simulink model "Banco_Capacitores_Automatico"  (R2022a)
settings: Solver=ode14x  StartTime=0.0  StopTime=1  FixedStep=5e-5  RelTol=1e-3
undefined symbols (not defined in the file): D11, Delta
libraries: spsSeriesRLCBranchLib x24, spsParallelRLCLoadLib x21, spsGroundLib x11, spsThreePhaseBreakerLib x7, spsLinearTransformerLib x6, spsCurrentMeasurementLib x4, spsVoltageMeasurementLib x3, eeRmsMeasurement x2, spsPower3phInstantaneousLib x2, spsThreePhaseVIMeasurementLib x2, spsThreePhaseSourceLib x1, spsRMSLib x1
settings Model: Creator=Luiz  LastModifiedBy=Luiz

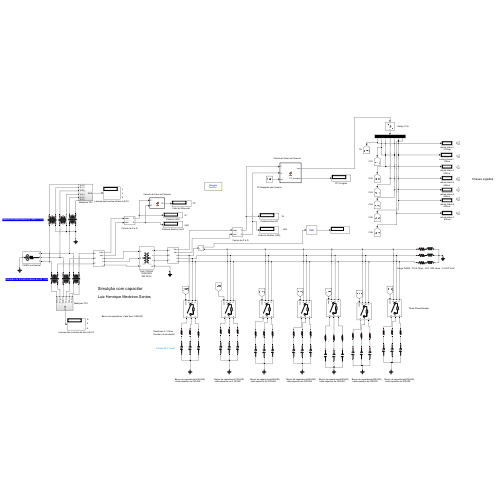
[thumbnail: Simulink's stored preview of the top-level diagram]
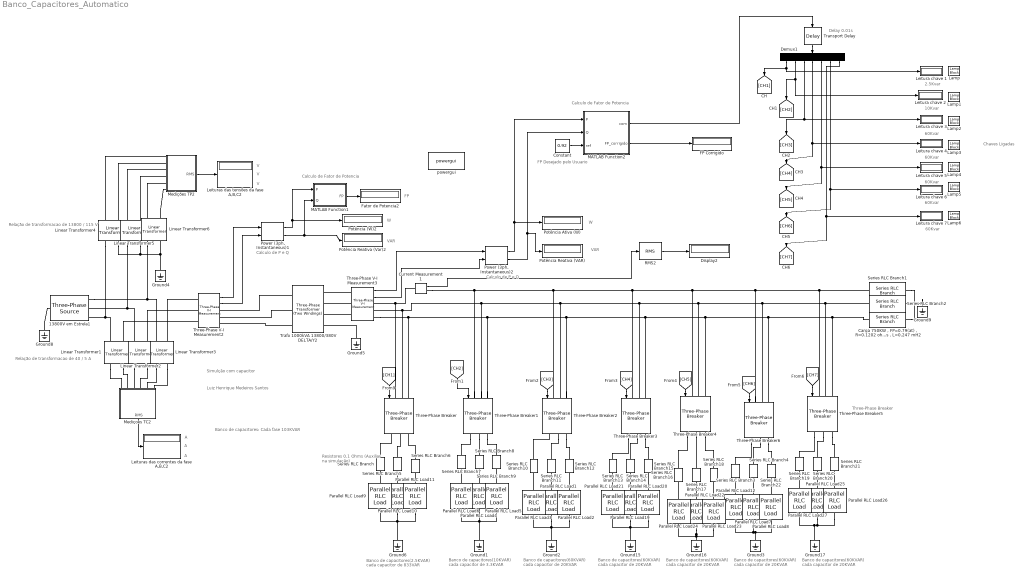
== system Banco_Capacitores_Automatico ==
  note: Three-Phase Breaker
  note: Banco de capacitores(2.5KVAR)
      |  cada capacitor de 833VAR
  note: Chaves Ligadas
  note: FP Desejado pelo Usuario
  note: 2.5Kvar
  note: Delay 0.01s
  note: Resistores 0.1 Ohms
      | (Auxiliar na simulação)
  note: A
  note: Simulção com capacitor
  note: Calculo de P e Q
  note: A
  note: V
  note: Luiz Henrique Medeiros Santos
  note: Relação de transformacao de 40 / 5 A
  note: V
  note: VAR
  note: FP
  note: Calculo de Fator de Potencia
  note: A
  note: V
  note: Calculo de P e Q
  note: Banco de capacitores: Cada fase 103KVAR
  note: VAR
  note: Relação de transformacao de 13800 / 115 V
  note: W
  note: Calculo de Fator de Potencia
  note: W
  note: 10Kvar
  note: 60Kvar
  note: 60Kvar
  note: 60Kvar
  note: 60Kvar
  note: 60Kvar
  note: Banco de capacitores(10KVAR)
      |  cada capacitor de 3.3KVAR
  note: Banco de capacitores(60KVAR)
      |  cada capacitor de 20KVAR
  note: Banco de capacitores(60KVAR)
      |  cada capacitor de 20KVAR
  note: Banco de capacitores(60KVAR)
      |  cada capacitor de 20KVAR
  note: Banco de capacitores(60KVAR)
      |  cada capacitor de 20KVAR
  note: Banco de capacitores(60KVAR)
      |  cada capacitor de 20KVAR
  13800V em Estrela1 : spsThreePhaseSourceLib/Three-Phase Source  InternalConnection=Yn  VoltagePhases=off  Voltage=13800  PhaseAngle=0  Voltage_phases=[25e3 25e3 25e3]/sqrt(3)  PhaseAngles_phases=[0 -120 +120]  Frequency=60  NonIdealSource=on  SpecifyImpedance=off  Resistance=0.0001  Inductance=0  ShortCircuitLevel=100e6  BaseVoltage=0  XRratio=7  BusType=swing  Pref=10e3  Qref=0  Prefabc=[10e3, 10e3, 10e3]  Qrefabc=[0, 0, 0]  Qmin=-inf  Qmax=inf
  "Carga 750KW , FP=0.79(at) , R=0.1202 ohms , L=0,247 mH2" : spsSeriesRLCBranchLib/Series RLC Branch  LConnTagsString=__new0  RConnTagsString=__new0  BranchType=RL  Resistance=0.1202  Inductance=0.247e-3  SetiL0=off  InitialCurrent=0  Capacitance=0  Setx0=off  InitialVoltage=0  Measurements=None
  Constant : Constant  Value=0.92
  Current Measurement1 : spsCurrentMeasurementLib/Current Measurement  PhasorSimulation=off  OutputType=Complex  PSBequivalent=0
  Demux1 : Demux  Outputs=7
  Display2 : Display
  FP Corrigido : Display
      settings: Format=bank
  Fator de Potencia2 : Display
      settings: Format=bank
  Ground{1..6,8..9,15..17} (11 alike) : spsGroundLib/Ground  LConnTagsString=a
  Lamp{,1..6} (7 alike) : LampBlock  LabelPosition=Hide
  Leitura chave {1..7} (7 alike) : Display
  Leituras das correntes da fase A,B,C2 : Display
      settings: Format=bank
  Leituras das tensões da fase A,B,C2 : Display
      settings: Format=bank
  Linear Transformer1 : spsLinearTransformerLib/Linear Transformer  UNITS=pu  NominalPower=[ 500 60 ]  winding1="[ 1 0.002  0.08 ]"  winding2="[ 8  0.002  0.08 ]"  ThreeWindings=off  winding3=[ 315e3 0.002 0.08 ]  RmLm=[ 500 500 ]  Measurements=None  DataType=off
  Linear Transformer2 : spsLinearTransformerLib/Linear Transformer  UNITS=pu  NominalPower=[ 500 60 ]  winding1="[ 1 0.002  0.08 ]"  winding2="[ 8  0.002  0.08 ]"  ThreeWindings=off  winding3=[ 315e3 0.002 0.08 ]  RmLm=[ 500 500 ]  Measurements=None  DataType=off
  Linear Transformer3 : spsLinearTransformerLib/Linear Transformer  UNITS=pu  NominalPower=[ 500 60 ]  winding1="[ 1 0.002  0.08 ]"  winding2="[ 8  0.002  0.08 ]"  ThreeWindings=off  winding3=[ 315e3 0.002 0.08 ]  RmLm=[ 500 500 ]  Measurements=None  DataType=off
  Linear Transformer4 : spsLinearTransformerLib/Linear Transformer  UNITS=pu  NominalPower=[ 500 60 ]  winding1="[ 7970 0.002  0.08 ]"  winding2="[ 115  0.002  0.08 ]"  ThreeWindings=off  winding3=[ 315e3 0.002 0.08 ]  RmLm=[ 500 500 ]  Measurements=None  DataType=off
  Linear Transformer5 : spsLinearTransformerLib/Linear Transformer  UNITS=pu  NominalPower=[ 500 60 ]  winding1="[ 7970 0.002  0.08 ]"  winding2="[ 115  0.002  0.08 ]"  ThreeWindings=off  winding3=[ 315e3 0.002 0.08 ]  RmLm=[ 500 500 ]  Measurements=None  DataType=off
  Linear Transformer6 : spsLinearTransformerLib/Linear Transformer  UNITS=pu  NominalPower=[ 500 60 ]  winding1="[ 7970 0.002  0.08 ]"  winding2="[ 115  0.002  0.08 ]"  ThreeWindings=off  winding3=[ 315e3 0.002 0.08 ]  RmLm=[ 500 500 ]  Measurements=None  DataType=off
  MATLAB Function1 : MATLAB Function  TreatAsAtomicUnit=on
  MATLAB Function2 : MATLAB Function  TreatAsAtomicUnit=on  SystemSampleTime=1
  Mediçoes TC2 : Subsystem
  Medições TP2 : Subsystem
  Parallel RLC Load{1,3,7..8,12,19..27} (14 alike) : spsParallelRLCLoadLib/Parallel RLC Load  LConnTagsString=a  RConnTagsString=__new0  NominalVoltage=217.78  NominalFrequency=60  ActivePower=0  InductivePower=0  CapacitivePower=20e3  Setx0=off  InitialVoltage=0  SetiL0=off  InitialCurrent=0  Measurements=None  LoadType=constant Z
      settings: AttributesFormatString=\n  SourceProductBaseCode=PS
  Parallel RLC Load10 : spsParallelRLCLoadLib/Parallel RLC Load  LConnTagsString=a  RConnTagsString=__new0  NominalVoltage=217.78  NominalFrequency=60  ActivePower=0  InductivePower=0  CapacitivePower=0.833e3  Setx0=off  InitialVoltage=0  SetiL0=off  InitialCurrent=0  Measurements=None  LoadType=constant Z
      settings: AttributesFormatString=\n  SourceProductBaseCode=PS
  Parallel RLC Load11 : spsParallelRLCLoadLib/Parallel RLC Load  LConnTagsString=a  RConnTagsString=__new0  NominalVoltage=217.78  NominalFrequency=60  ActivePower=0  InductivePower=0  CapacitivePower=0.833e3  Setx0=off  InitialVoltage=0  SetiL0=off  InitialCurrent=0  Measurements=None  LoadType=constant Z
      settings: AttributesFormatString=\n  SourceProductBaseCode=PS
  Parallel RLC Load2 : spsParallelRLCLoadLib/Parallel RLC Load  LConnTagsString=a  RConnTagsString=__new0  NominalVoltage=217.78  NominalFrequency=60  ActivePower=0  InductivePower=0  CapacitivePower=20e3  Setx0=off  InitialVoltage=0  SetiL0=on  InitialCurrent=0  Measurements=None  LoadType=constant Z
      settings: AttributesFormatString=\n  SourceProductBaseCode=PS
  Parallel RLC Load4 : spsParallelRLCLoadLib/Parallel RLC Load  LConnTagsString=a  RConnTagsString=__new0  NominalVoltage=217.78  NominalFrequency=60  ActivePower=0  InductivePower=0  CapacitivePower=3.33e3  Setx0=off  InitialVoltage=0  SetiL0=off  InitialCurrent=0  Measurements=None  LoadType=constant Z
      settings: AttributesFormatString=\n  SourceProductBaseCode=PS
  Parallel RLC Load5 : spsParallelRLCLoadLib/Parallel RLC Load  LConnTagsString=a  RConnTagsString=__new0  NominalVoltage=217.78  NominalFrequency=60  ActivePower=0  InductivePower=0  CapacitivePower=3.33e3  Setx0=off  InitialVoltage=0  SetiL0=off  InitialCurrent=0  Measurements=None  LoadType=constant Z
      settings: AttributesFormatString=\n  SourceProductBaseCode=PS
  Parallel RLC Load6 : spsParallelRLCLoadLib/Parallel RLC Load  LConnTagsString=a  RConnTagsString=__new0  NominalVoltage=217.78  NominalFrequency=60  ActivePower=0  InductivePower=0  CapacitivePower=3.33e3  Setx0=off  InitialVoltage=0  SetiL0=off  InitialCurrent=0  Measurements=None  LoadType=constant Z
      settings: AttributesFormatString=\n  SourceProductBaseCode=PS
  Parallel RLC Load9 : spsParallelRLCLoadLib/Parallel RLC Load  LConnTagsString=a  RConnTagsString=__new0  NominalVoltage=217.78  NominalFrequency=60  ActivePower=0  InductivePower=0  CapacitivePower=0.833e3  Setx0=off  InitialVoltage=0  SetiL0=off  InitialCurrent=0  Measurements=None  LoadType=constant Z
      settings: AttributesFormatString=\n  SourceProductBaseCode=PS
  Potência (W)2 : Display
      settings: Format=bank
  Potência Ativa (W) : Display
      settings: Format=bank
  Potência Reativa (VAR) : Display
      settings: Format=bank
  Potência Reativa (Var)2 : Display
      settings: Format=bank
  "Power (3ph, Instantaneous)1" : spsPower3phInstantaneousLib/Power (3ph, Instantaneous)
  "Power (3ph, Instantaneous)2" : spsPower3phInstantaneousLib/Power (3ph, Instantaneous)
  RMS2 : spsRMSLib/RMS  TrueRMS=on  Freq=60  RMSInit=120  Ts=0
  Series RLC Branch{,3..22} (21 alike) : spsSeriesRLCBranchLib/Series RLC Branch  LConnTagsString=__new0  RConnTagsString=__new0  BranchType=R  Resistance=0.05  Inductance=0  SetiL0=off  InitialCurrent=0  Capacitance=0  Setx0=off  InitialVoltage=0  Measurements=None
  Series RLC Branch1 : spsSeriesRLCBranchLib/Series RLC Branch  LConnTagsString=__new0  RConnTagsString=__new0  BranchType=RL  Resistance=0.1202  Inductance=0.247e-3  SetiL0=off  InitialCurrent=0  Capacitance=0  Setx0=off  InitialVoltage=0  Measurements=None
  Series RLC Branch2 : spsSeriesRLCBranchLib/Series RLC Branch  LConnTagsString=__new0  RConnTagsString=__new0  BranchType=RL  Resistance=0.1202  Inductance=0.247e-3  SetiL0=off  InitialCurrent=0  Capacitance=0  Setx0=off  InitialVoltage=0  Measurements=None
  Three-Phase V-I Measurement2 : spsThreePhaseVIMeasurementLib/Three-Phase V-I Measurement  VoltageMeasurement=phase-to-ground  SetLabelV=off  LabelV=Vabc  Vpu=off  VpuLL=off  CurrentMeasurement=yes  SetLabelI=off  LabelI=Iabc  Ipu=off  Pbase=100e6  Vbase=500e3  OutputType=Complex  PhasorSimulation=off  PSBequivalent=0
  Three-Phase V-I Measurement3 : spsThreePhaseVIMeasurementLib/Three-Phase V-I Measurement  VoltageMeasurement=phase-to-ground  SetLabelV=off  LabelV=Vabc  Vpu=off  VpuLL=off  CurrentMeasurement=yes  SetLabelI=off  LabelI=Iabc  Ipu=off  Pbase=100e6  Vbase=500e3  OutputType=Complex  PhasorSimulation=off  PSBequivalent=0
  Three-Phase Breaker{,1..6} (7 alike) : spsThreePhaseBreakerLib/Three-Phase Breaker  InitialState=open  SwitchA=on  SwitchB=on  SwitchC=on  SwitchTimes="[1/60  5/60]"  External=on  BreakerResistance=0.01  SnubberResistance=1e6  SnubberCapacitance=inf  Measurements=None
  Trafo 1000kVA 13800/380V DELTA/Y2 : spsThreePhaseTransformerTwoWindingsLib/Three-Phase Transformer (Two Windings)  Winding1Connection=Delta (D11)  Winding2Connection=Yn  CoreType=Three single-phase transformers  SetSaturation=off  Hysteresis=off  DataFile='hysteresis'  SetInitialFlux=off  Measurements=None  UNITS=SI  NominalPower=[ 1e6 , 60 ]  Winding1=[13800 0.0001 0.0001]  Winding2=[380 0.00001 1e-05]  Rm=2.8566e+06  Lm=757.74  L0=0.5  Saturation=[0 0;0.081983 62.122;34.16 78.688]  InitialFluxes=[ 0.8 , -0.8 , 0.7 ]  BreakLoop=off  DiscreteSolver=Trapezoidal iterative  DataType=on  TransfoNumber=1
  Transport Delay : TransportDelay  DelayTime=0.1  BufferSize=10240
  powergui : spspowerguiLib/powergui  Priority=1  SimulationMode=Discrete  SampleTime=50e-6  frequency=60  Iterations=50  frequencyindice=60  Pbase=100e6  ErrMax=1e-4  UnitsV=kV  UnitsW=MW  buscounter=0  FunctionMessages=off  echomessages=off  EnableUseOfTLC=off  CurrentSourceSwitches=off  DisableSnubberDevices=off  DisableRonSwitches=off  DisableVfSwitches=off  DisplayEquations=off  AutomaticDiscreteSolvers=off  SolverType=Tustin/Backward Euler (TBE)  Interpol=off  ExternalGateDelay=off  methode=off  Ts=100  x0status=blocks  SPID=on  SwTol=0  HookPort=off  NonlinearTolerance=1e-4  nMaxIteration=100  ContinueOnMaxIteration=off  RestoreLinks=warning  ResistiveCurrentMeasurement=off  Frange=[0:2:500]  Ylog=off  Xlog=on  ShowGrid=off  save=off  variable=ZData  structure=0  ZoomFFT=off  StartTime=0.0  cycles=1  DisplayStyle=1  fundamental=60  FreqAxis=off  MaxFrequency=1000  frequencyindicesteady=1  RmsSteady=1  display=off
  wires:
  "Power (3ph, Instantaneous)1"/1 -> MATLAB Function1/1(P), Potência (W)2/1
  Three-Phase V-I Measurement2/1 -> "Power (3ph, Instantaneous)1"/1
  Mediçoes TC2/1(RMS) -> Leituras das correntes da fase A,B,C2/1
  "Power (3ph, Instantaneous)1"/2 -> MATLAB Function1/2(Q), Potência Reativa (Var)2/1
  Three-Phase V-I Measurement3/2 -> "Power (3ph, Instantaneous)2"/2
  Current Measurement1/1 -> RMS2/1
  "Power (3ph, Instantaneous)2"/2 -> MATLAB Function2/2(Q), Potência Reativa (VAR)/1
  RMS2/1 -> Display2/1
  MATLAB Function2/2(FP_corrigido) -> FP Corrigido/1
  MATLAB Function1/1(FP) -> Fator de Potencia2/1
  Three-Phase V-I Measurement3/1 -> "Power (3ph, Instantaneous)2"/1
  Medições TP2/1(RMS) -> Leituras das tensões da fase A,B,C2/1
  "Power (3ph, Instantaneous)2"/1 -> MATLAB Function2/1(P), Potência Ativa (W)/1
  MATLAB Function2/1(com) -> Transport Delay/1
  Three-Phase V-I Measurement2/2 -> "Power (3ph, Instantaneous)1"/2
  Demux1/1 -> Leitura chave 1/1, [CH1]
  Demux1/2 -> Leitura chave 2/1, [CH2]
  Demux1/3 -> Leitura chave 3/1, [CH3]
  Demux1/4 -> [CH4], Leitura chave 4/1
  Demux1/5 -> [CH5], Leitura chave 5/1
  Demux1/6 -> [CH6], Leitura chave 6/1
  Demux1/7 -> [CH7], Leitura chave 7/1
  Constant/1 -> MATLAB Function2/3(ref)
  Transport Delay/1 -> Demux1/1
  [CH2] -> Three-Phase Breaker1/1
  [CH3] -> Three-Phase Breaker2/1
  [CH4] -> Three-Phase Breaker3/1
  [CH5] -> Three-Phase Breaker4/1
  [CH6] -> Three-Phase Breaker6/1
  [CH7] -> Three-Phase Breaker5/1
  [CH1] -> Three-Phase Breaker/1
  connections:
  Linear Transformer6/LConn1 -- Linear Transformer3/LConn1 -- 13800V em Estrela1/RConn1
  Linear Transformer2/LConn1 -- 13800V em Estrela1/RConn2 -- Linear Transformer5/LConn1
  Current Measurement1/LConn1 -- Three-Phase V-I Measurement3/RConn1 -- Three-Phase Breaker/LConn1
  Ground4/LConn1 -- Linear Transformer6/LConn2 -- Linear Transformer4/LConn2 -- Linear Transformer5/LConn2
  Series RLC Branch2/LConn1 -- Three-Phase Breaker6/LConn2 -- Three-Phase Breaker4/LConn2 -- Three-Phase Breaker3/LConn2 -- Three-Phase Breaker1/LConn2 -- Three-Phase V-I Measurement3/RConn2 -- Three-Phase Breaker/LConn2 -- Three-Phase Breaker2/LConn2 -- Three-Phase Breaker5/LConn2
  Parallel RLC Load9/RConn1 -- Parallel RLC Load11/RConn1 -- Ground6/LConn1 -- Parallel RLC Load10/RConn1
  Three-Phase V-I Measurement3/RConn3 -- Three-Phase Breaker1/LConn3 -- Three-Phase Breaker2/LConn3 -- Three-Phase Breaker3/LConn3 -- Three-Phase Breaker4/LConn3 -- Three-Phase Breaker6/LConn3 -- Three-Phase Breaker5/LConn3 -- "Carga 750KW , FP=0.79(at) , R=0.1202 ohms , L=0,247 mH2"/LConn1 -- Three-Phase Breaker/LConn3
  Linear Transformer4/LConn1 -- 13800V em Estrela1/RConn3 -- Linear Transformer1/LConn1
  Current Measurement1/RConn1 -- Three-Phase Breaker1/LConn1 -- Three-Phase Breaker3/LConn1 -- Three-Phase Breaker4/LConn1 -- Three-Phase Breaker6/LConn1 -- Three-Phase Breaker5/LConn1 -- Series RLC Branch1/LConn1 -- Three-Phase Breaker2/LConn1
  Three-Phase V-I Measurement3/LConn2 -- Trafo 1000kVA 13800/380V DELTA/Y2/RConn2
  Linear Transformer3/LConn2 -- Three-Phase V-I Measurement2/LConn1
  Three-Phase V-I Measurement3/LConn3 -- Trafo 1000kVA 13800/380V DELTA/Y2/RConn3
  Linear Transformer6/RConn2 -- Medições TP2/LConn6
  Ground8/LConn1 -- 13800V em Estrela1/LConn1
  Parallel RLC Load9/LConn1 -- Series RLC Branch/RConn1
  Trafo 1000kVA 13800/380V DELTA/Y2/LConn3 -- Three-Phase V-I Measurement2/RConn3
  Linear Transformer5/RConn2 -- Medições TP2/LConn4
  Linear Transformer2/RConn1 -- Mediçoes TC2/LConn3
  Linear Transformer6/RConn1 -- Medições TP2/LConn5
  Linear Transformer1/RConn1 -- Mediçoes TC2/LConn1
  Linear Transformer3/RConn2 -- Mediçoes TC2/LConn6
  Linear Transformer4/RConn2 -- Medições TP2/LConn2
  Trafo 1000kVA 13800/380V DELTA/Y2/LConn2 -- Three-Phase V-I Measurement2/RConn2
  Three-Phase V-I Measurement3/LConn1 -- Trafo 1000kVA 13800/380V DELTA/Y2/RConn1
  Trafo 1000kVA 13800/380V DELTA/Y2/LConn1 -- Three-Phase V-I Measurement2/RConn1
  Linear Transformer2/LConn2 -- Three-Phase V-I Measurement2/LConn2
  Parallel RLC Load10/LConn1 -- Series RLC Branch5/RConn1
  Linear Transformer1/RConn2 -- Mediçoes TC2/LConn2
  Linear Transformer3/RConn1 -- Mediçoes TC2/LConn5
  Linear Transformer5/RConn1 -- Medições TP2/LConn3
  Linear Transformer2/RConn2 -- Mediçoes TC2/LConn4
  Linear Transformer4/RConn1 -- Medições TP2/LConn1
  Linear Transformer1/LConn2 -- Three-Phase V-I Measurement2/LConn3
  Ground5/LConn1 -- Trafo 1000kVA 13800/380V DELTA/Y2/RConn4
  Series RLC Branch6/LConn1 -- Three-Phase Breaker/RConn3
  Ground9/LConn1 -- "Carga 750KW , FP=0.79(at) , R=0.1202 ohms , L=0,247 mH2"/RConn1 -- Series RLC Branch1/RConn1 -- Series RLC Branch2/RConn1
  Parallel RLC Load4/RConn1 -- Parallel RLC Load5/RConn1 -- Ground1/LConn1 -- Parallel RLC Load6/RConn1
  Parallel RLC Load4/LConn1 -- Series RLC Branch8/RConn1
  Parallel RLC Load6/LConn1 -- Series RLC Branch7/RConn1
  Parallel RLC Load5/LConn1 -- Series RLC Branch9/RConn1
  Parallel RLC Load1/RConn1 -- Parallel RLC Load2/RConn1 -- Ground2/LConn1 -- Parallel RLC Load3/RConn1
  Parallel RLC Load2/LConn1 -- Series RLC Branch12/RConn1
  Parallel RLC Load3/LConn1 -- Series RLC Branch10/RConn1
  Parallel RLC Load1/LConn1 -- Series RLC Branch11/RConn1
  Series RLC Branch/LConn1 -- Three-Phase Breaker/RConn1
  Series RLC Branch5/LConn1 -- Three-Phase Breaker/RConn2
  Parallel RLC Load11/LConn1 -- Series RLC Branch6/RConn1
  Three-Phase Breaker1/RConn1 -- Series RLC Branch7/LConn1
  Three-Phase Breaker1/RConn2 -- Series RLC Branch8/LConn1
  Three-Phase Breaker1/RConn3 -- Series RLC Branch9/LConn1
  Three-Phase Breaker2/RConn1 -- Series RLC Branch10/LConn1
  Three-Phase Breaker2/RConn2 -- Series RLC Branch11/LConn1
  Three-Phase Breaker2/RConn3 -- Series RLC Branch12/LConn1
  Parallel RLC Load21/RConn1 -- Parallel RLC Load19/RConn1 -- Parallel RLC Load20/RConn1 -- Ground15/LConn1
  Three-Phase Breaker3/RConn2 -- Series RLC Branch14/LConn1
  Three-Phase Breaker3/RConn1 -- Series RLC Branch13/LConn1
  Parallel RLC Load21/LConn1 -- Series RLC Branch13/RConn1
  Three-Phase Breaker3/RConn3 -- Series RLC Branch15/LConn1
  Parallel RLC Load19/LConn1 -- Series RLC Branch14/RConn1
  Parallel RLC Load20/LConn1 -- Series RLC Branch15/RConn1
  Parallel RLC Load24/RConn1 -- Parallel RLC Load22/RConn1 -- Ground16/LConn1 -- Parallel RLC Load23/RConn1
  Three-Phase Breaker4/RConn2 -- Series RLC Branch17/LConn1
  Three-Phase Breaker4/RConn1 -- Series RLC Branch16/LConn1
  Parallel RLC Load24/LConn1 -- Series RLC Branch16/RConn1
  Three-Phase Breaker4/RConn3 -- Series RLC Branch18/LConn1
  Parallel RLC Load22/LConn1 -- Series RLC Branch17/RConn1
  Parallel RLC Load23/LConn1 -- Series RLC Branch18/RConn1
  Parallel RLC Load27/RConn1 -- Parallel RLC Load25/RConn1 -- Parallel RLC Load26/RConn1 -- Ground17/LConn1
  Three-Phase Breaker5/RConn2 -- Series RLC Branch20/LConn1
  Three-Phase Breaker5/RConn1 -- Series RLC Branch19/LConn1
  Parallel RLC Load27/LConn1 -- Series RLC Branch19/RConn1
  Three-Phase Breaker5/RConn3 -- Series RLC Branch21/LConn1
  Parallel RLC Load25/LConn1 -- Series RLC Branch20/RConn1
  Parallel RLC Load26/LConn1 -- Series RLC Branch21/RConn1
  Parallel RLC Load12/RConn1 -- Parallel RLC Load8/RConn1 -- Ground3/LConn1 -- Parallel RLC Load7/RConn1
  Three-Phase Breaker6/RConn2 -- Series RLC Branch4/LConn1
  Three-Phase Breaker6/RConn1 -- Series RLC Branch3/LConn1
  Parallel RLC Load12/LConn1 -- Series RLC Branch3/RConn1
  Three-Phase Breaker6/RConn3 -- Series RLC Branch22/LConn1
  Parallel RLC Load7/LConn1 -- Series RLC Branch4/RConn1
  Parallel RLC Load8/LConn1 -- Series RLC Branch22/RConn1

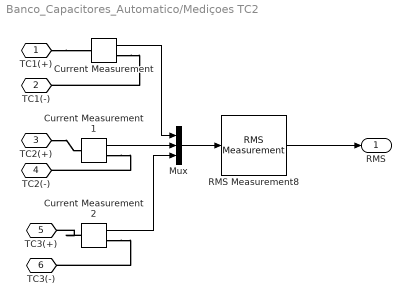
== system Banco_Capacitores_Automatico/Mediçoes TC2 ==
  Current Measurement : spsCurrentMeasurementLib/Current Measurement  PhasorSimulation=off  OutputType=Complex  PSBequivalent=0
  Current Measurement1 : spsCurrentMeasurementLib/Current Measurement  PhasorSimulation=off  OutputType=Complex  PSBequivalent=0
  Current Measurement2 : spsCurrentMeasurementLib/Current Measurement  PhasorSimulation=off  OutputType=Complex  PSBequivalent=0
  Mux : Mux  Inputs=3
  RMS Measurement8 : eeRmsMeasurement/RMS Measurement  LabelModeActiveChoice=Total  F=60  SpecifyHarmonics=off  K=[0 1 2]  Ts=0
      settings: SourceProductBaseCode=PS
  TC1(+) : PMIOPort  Side=Left
  TC1(-) : PMIOPort  Port=2  Side=Left
  TC2(+) : PMIOPort  Port=3  Side=Left
  TC2(-) : PMIOPort  Port=4  Side=Left
  TC3(+) : PMIOPort  Port=5  Side=Left
  TC3(-) : PMIOPort  Port=6  Side=Left
  RMS : Outport
  wires:
  RMS Measurement8/1 -> RMS/1
  Current Measurement/1 -> Mux/1
  Mux/1 -> RMS Measurement8/1
  Current Measurement2/1 -> Mux/3
  Current Measurement1/1 -> Mux/2
  connections:
  Current Measurement/RConn1 -- TC1(-)/RConn1
  TC1(+)/RConn1 -- Current Measurement/LConn1
  TC2(+)/RConn1 -- Current Measurement1/LConn1
  Current Measurement1/RConn1 -- TC2(-)/RConn1
  Current Measurement2/LConn1 -- TC3(+)/RConn1
  Current Measurement2/RConn1 -- TC3(-)/RConn1

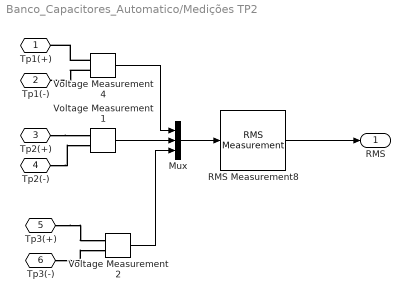
== system Banco_Capacitores_Automatico/Medições TP2 ==
  Mux : Mux  Inputs=3
  RMS Measurement8 : eeRmsMeasurement/RMS Measurement  LabelModeActiveChoice=Total  F=60  SpecifyHarmonics=off  K=[0 1 2]  Ts=0
      settings: SourceProductBaseCode=PS
  Voltage Measurement1 : spsVoltageMeasurementLib/Voltage Measurement  PhasorSimulation=off  OutputType=Complex  PSBequivalent=0
  Voltage Measurement2 : spsVoltageMeasurementLib/Voltage Measurement  PhasorSimulation=off  OutputType=Complex  PSBequivalent=0
  Voltage Measurement4 : spsVoltageMeasurementLib/Voltage Measurement  PhasorSimulation=off  OutputType=Complex  PSBequivalent=0
  Tp1(+) : PMIOPort  Side=Left
  Tp1(-) : PMIOPort  Port=2  Side=Left
  Tp2(+) : PMIOPort  Port=3  Side=Left
  Tp2(-) : PMIOPort  Port=4  Side=Left
  Tp3(+) : PMIOPort  Port=5  Side=Left
  Tp3(-) : PMIOPort  Port=6  Side=Left
  RMS : Outport
  wires:
  RMS Measurement8/1 -> RMS/1
  Voltage Measurement4/1 -> Mux/1
  Voltage Measurement1/1 -> Mux/2
  Voltage Measurement2/1 -> Mux/3
  Mux/1 -> RMS Measurement8/1
  connections:
  Voltage Measurement4/LConn2 -- Tp1(-)/RConn1
  Voltage Measurement4/LConn1 -- Tp1(+)/RConn1
  Tp2(+)/RConn1 -- Voltage Measurement1/LConn1
  Tp2(-)/RConn1 -- Voltage Measurement1/LConn2
  Tp3(+)/RConn1 -- Voltage Measurement2/LConn1
  Tp3(-)/RConn1 -- Voltage Measurement2/LConn2

== matlab function Banco_Capacitores_Automatico/MATLAB Function1 ==
  data: P input; FP output; Q input
function FP = fcn(P,Q)

p=P^2;

q=Q^2;

FP= P/(sqrt(p+q));

== matlab function Banco_Capacitores_Automatico/MATLAB Function2 ==
  data: com output; P input; FP_corrigido output; Q input; ref input
function [com,FP_corrigido] = fcn(P, Q, ref)

% Memória para guardar o estado das chaves
persistent estado
if isempty(estado)
    estado = zeros(1,7); % Ajustado para 7 chaves
end


% --- Trava de Segurança Inicial ---


% --- Parâmetros Físicos Atualizados ---
% Vetor ordenado do MAIOR para o MENOR para ajuste inteligente
Banco = [2.5e3, 10e3, 60e3, 60e3, 60e3, 60e3 ,60e3 ];

liga = estado;
soma = sum(liga .* Banco);

% Estimativa da Carga Real
Q_carga = Q + soma;
Q_alvo = P * tan(acos(ref));
Qdsj = Q_carga - Q_alvo;

if Qdsj < 0
    Qdsj = 0;
end

% --- LÓGICA DE LIGAÇÃO (Testa os maiores degraus primeiro) ---
for t = 1:length(Banco)
    % A margem agora é dinâmica: 55% do tamanho do estágio avaliado
    margem_dinamica = Banco(t) * 0.6; 
    
    if soma < (Qdsj - margem_dinamica) && liga(t) == 0
        soma = soma + Banco(t);
        liga(t) = 1;
    end
end

% --- LÓGICA DE DESLIGAMENTO (Testa os menores degraus primeiro) ---
for t = length(Banco):-1:1
    margem_dinamica = Banco(t) * 0.55;
    
    if soma > (Qdsj + margem_dinamica) && liga(t) == 1
        soma = soma - Banco(t);
        liga(t) = 0;
    end
end

% Atualização de Memória
estado = liga;
com = liga'; % Saída de 7 vias

% Cálculo do FP estimado
Q_rede_estimado = Q_carga - soma; 
S_estimado = sqrt(P^2 + Q_rede_estimado^2);
if S_estimado > 0
    FP_corrigido = P / S_estimado;
else
    FP_corrigido = 1;
end


end
